simulink model "simrf_noise_source"  (R2015a)
settings: Solver=VariableStepDiscrete  StartTime=0.0  StopTime=0.1  RelTol=1e-3
PreLoadFcn:
  | k = 1.38065e-23;
  | R = 50;
  | Freq = 2e9;
  | time_step = 1e-6;
values from neighbouring files (symbols this model uses):
  kb = 1.38e-23    [noise_source_runcfg.m]
  Rnoise = 620+200    (= 820)    [noise_source_runcfg.m]
libraries: simrfV2util1 x2, simrfV2sources1 x1, fl_lib x1, simrfV2elements x1
CloseFcn:
  | clear k R Freq time_step
settings Model: FPTRunName=Active  Creator=The MathWorks Inc.  LastModifiedBy=mainster
settings OptimizationCC: ExpressionDepthLimit=2147483647
settings DebuggingCC: UnderspecifiedInitializationDetection=Classic  MergeDetectMultiDrivingBlocksExec=none  SolverPrmCheckMsg=warning  FcnCallInpInsideContextMsg=UseLocalSettings  StateNameClashWarn=warning
settings GRTTargetCC: CombineOutputUpdateFcns=off  GRTInterface=on

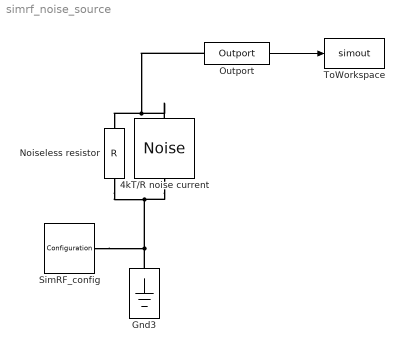
== system simrf_noise_source ==
  4kT/R noise current : simrfV2sources1/Noise  SimulinkInputSignalType=Ideal current  NoiseType=White  NoisePSD=4*kb*293/Rnoise  CarrierFreq=0 Hz  InternalGrounding=off
  Gnd3 : fl_lib/Electrical/Electrical Elements/Electrical Reference
  Noiseless resistor : simrfV2elements/R  classname=resistor  Resistance=Rnoise Ohm  AddNoise=off
  Outport : simrfV2util1/Outport  SensorType=Ideal voltage  OutputFormat=Real Passband  CarrierFreq=0 Hz  ZL=Inf  InternalGrounding=on  StepSize=-1 s  AutoStep=off
  SimRF_config : simrfV2util1/Configuration  AutoFreq=on  Tones=[2] GHz  Harmonics=[7]  NormalizeCarrierPower=off  SolverType=Auto  StepSize=3.9063e-06 s  AddNoise=on  Temperature=273+20 K  SolverDelFlag=0
  ToWorkspace : ToWorkspace  VariableName=simout  SaveFormat=Timeseries  SampleTime=-1
  wires:
  Outport/1 -> ToWorkspace/1
  connections:
  Gnd3/LConn1 -- 4kT/R noise current/RConn1 -- Noiseless resistor/RConn1 -- SimRF_config/LConn1
  4kT/R noise current/LConn1 -- Outport/LConn1 -- Noiseless resistor/LConn1
